simulink model "homework3_simulation"  (R2021a)
settings: Solver=VariableStepAuto  StartTime=0.0  StopTime=18  RelTol=1e-3
values from neighbouring files (symbols this model uses):
  Caf = 10000    [Homework3.m]
  Car = 10000    [Homework3.m]
  F1 = Ys1 * inv(Xs)    [Homework3.m]
  F2 = Ys2 * inv(Xs)    [Homework3.m]
  Iz = 50000    [Homework3.m]
  lf = 1.4    [Homework3.m]
  lr = 1.4    [Homework3.m]
  m = 1800    [Homework3.m]
settings Model: Creator=seo27  LastModifiedBy=seo27
settings SolverCC: AlgebraicLoopSolver=LineSearch
settings DebuggingCC: SFMachineParentedDataDiag=warning

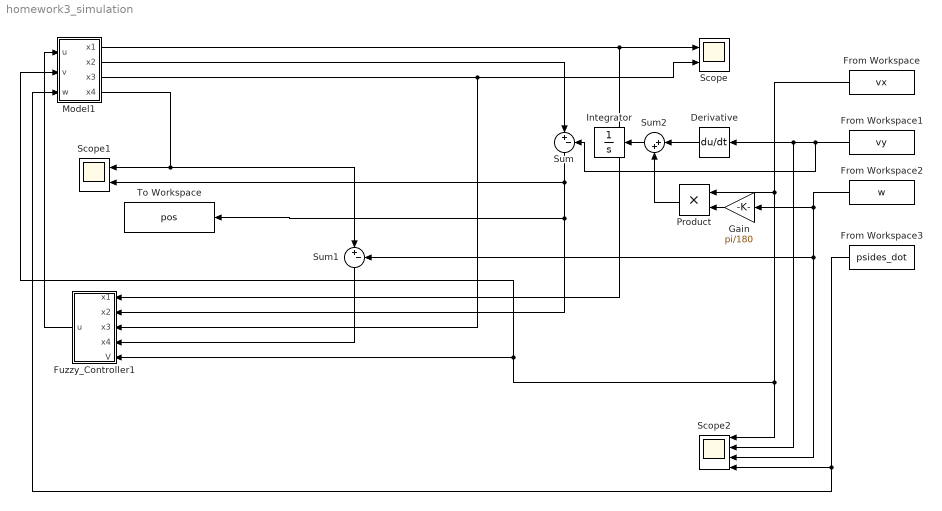
== system homework3_simulation ==
  Derivative : Derivative  CoefficientInTFapproximation=0.02
  From Workspace : FromWorkspace  VariableName=vx  SampleTime=0.02
  From Workspace1 : FromWorkspace  VariableName=vy  SampleTime=0.02
  From Workspace2 : FromWorkspace  VariableName=w  SampleTime=0.02
  From Workspace3 : FromWorkspace  VariableName=psides_dot  SampleTime=0.02
  Fuzzy_Controller1 : Subsystem
  Gain : Gain  Gain=pi/180
  Integrator : Integrator
  Model1 : Subsystem
  Product : Product
  Scope : Scope  NumInputPorts=2
  Scope1 : Scope  NumInputPorts=2
  Scope2 : Scope  NumInputPorts=4
  Sum : Sum  Inputs=|+-
  Sum1 : Sum  Inputs=|+-
  Sum2 : Sum  Inputs=|++
  To Workspace : ToWorkspace  VariableName=pos  SaveFormat=Structure With Time  SampleTime=0.02
  wires:
  Fuzzy_Controller1/1(u) -> Model1/1(u)
  From Workspace/1 -> Product/1, Scope2/1, Fuzzy_Controller1/5(V), Model1/2(v)
  Sum/1 -> Scope1/2, To Workspace/1, Fuzzy_Controller1/2(x2)
  Model1/2(x2) -> Sum/1
  Sum1/1 -> Fuzzy_Controller1/4(x4)
  Model1/4(x4) -> Sum1/1, Scope1/1
  Model1/3(x3) -> Fuzzy_Controller1/3(x3), Scope/2
  Model1/1(x1) -> Fuzzy_Controller1/1(x1), Scope/1
  From Workspace1/1 -> Sum/2, Scope2/2, Derivative/1
  Derivative/1 -> Sum2/1
  Product/1 -> Sum2/2
  Sum2/1 -> Integrator/1
  Gain/1 -> Product/2
  From Workspace2/1 -> Gain/1, Sum1/2, Scope2/3
  From Workspace3/1 -> Scope2/4, Model1/3(w)

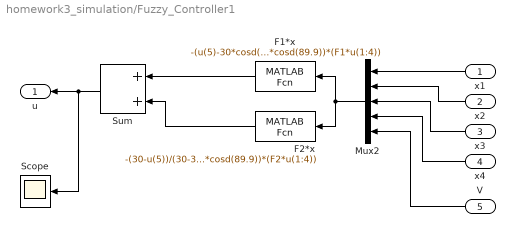
== system homework3_simulation/Fuzzy_Controller1 ==
  x1 : Inport
  x2 : Inport  Port=2
  x3 : Inport  Port=3
  x4 : Inport  Port=4
  V : Inport  Port=5
  F1*x : MATLABFcn  MATLABFcn=-(u(5)-30*cosd(89.9))/(30-30*cosd(89.9))*(F1*u(1:4))
  F2*x : MATLABFcn  MATLABFcn=-(30-u(5))/(30-30*cosd(89.9))*(F2*u(1:4))
  Mux2 : Mux  Inputs=5
  Scope : Scope
  Sum : Sum
  u : Outport
  wires:
  Sum/1 -> Scope/1, u/1
  x1/1 -> Mux2/1
  Mux2/1 -> F1*x/1, F2*x/1
  F1*x/1 -> Sum/1
  F2*x/1 -> Sum/2
  x3/1 -> Mux2/3
  x4/1 -> Mux2/4
  x2/1 -> Mux2/2
  V/1 -> Mux2/5

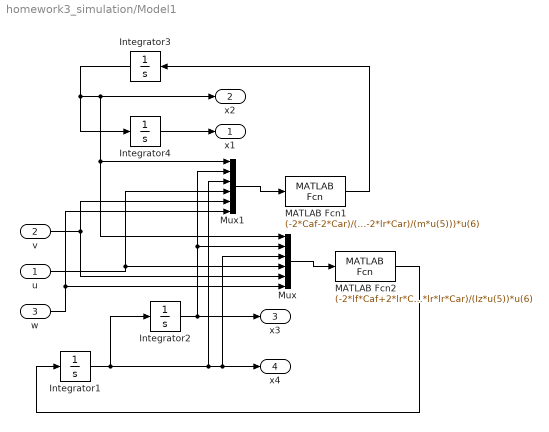
== system homework3_simulation/Model1 ==
  u : Inport
  v : Inport  Port=2
  w : Inport  Port=3
  Integrator1 : Integrator
  Integrator2 : Integrator
  Integrator3 : Integrator
  Integrator4 : Integrator  InitialCondition=1.35
  MATLAB Fcn1 : MATLABFcn  MATLABFcn=(-2*Caf-2*Car)/(m*u(5))*u(1)+(2*Caf+2*Car)/m*u(2)+(-2*lf*Caf+2*lr*Car)/(m*u(5))*u(3)+2*Caf/m*u(4)+(-u(5)-(2*lf*Caf-2*lr*Car)/(m*u(5)))*u(6)
  MATLAB Fcn2 : MATLABFcn  MATLABFcn=(-2*lf*Caf+2*lr*Car)/(Iz*u(5))*u(1)+(2*lf*Caf-2*lr*Car)/Iz*u(2)+(-2*lf*lf*Caf-2*lr*lr*Car)/(Iz*u(5))*u(3)+2*lf*Caf/Iz*u(4)-(2*lf*lf*Caf+2*lr*lr*Car)/(Iz*u(5))*u(6)
  Mux : Mux  Inputs=6
  Mux1 : Mux  Inputs=6
  x1 : Outport
  x2 : Outport  Port=2
  x3 : Outport  Port=3
  x4 : Outport  Port=4
  wires:
  Mux1/1 -> MATLAB Fcn1/1
  MATLAB Fcn1/1 -> Integrator3/1
  Mux/1 -> MATLAB Fcn2/1
  Integrator3/1 -> Mux/1, Mux1/1, x2/1, Integrator4/1
  Integrator4/1 -> x1/1
  Integrator2/1 -> Mux1/2, Mux/2, x3/1
  Integrator1/1 -> Integrator2/1, Mux1/3, Mux/3, x4/1
  MATLAB Fcn2/1 -> Integrator1/1
  u/1 -> Mux1/4, Mux/4
  v/1 -> Mux1/5, Mux/5
  w/1 -> Mux/6, Mux1/6
